simulink model "tanks_with_costate_equations_model"  (R2014a)
settings: Solver=ode4  StartTime=0.0  StopTime=T  FixedStep=0.001  RelTol=1e-3
values from neighbouring files (symbols this model uses):
  a = 31    [tanks_runner.m]
  b = 40    [tanks_runner.m]
  c = 10    [tanks_runner.m]
  C1 = 25    [tanks_runner.m]
  C2 = 25    [tanks_runner.m]
  C3 = 25    [tanks_runner.m]
  h10 = 10    [tanks_runner.m]
  h20 = 10    [tanks_runner.m]
  h30 = 10    [tanks_runner.m]
  h_max = 40    [tanks_runner.m]
  p = [sin(theta)*cos(phi); sin(theta)*sin(phi); cos(theta)]    [tanks_reachability_set.m]
  R = 40    [tanks_runner.m]
  u_max = 200    [tanks_runner.m]
  w = 5    [tanks_runner.m]
settings Model: Creator=Lukasz  LastModifiedBy=Lukasz

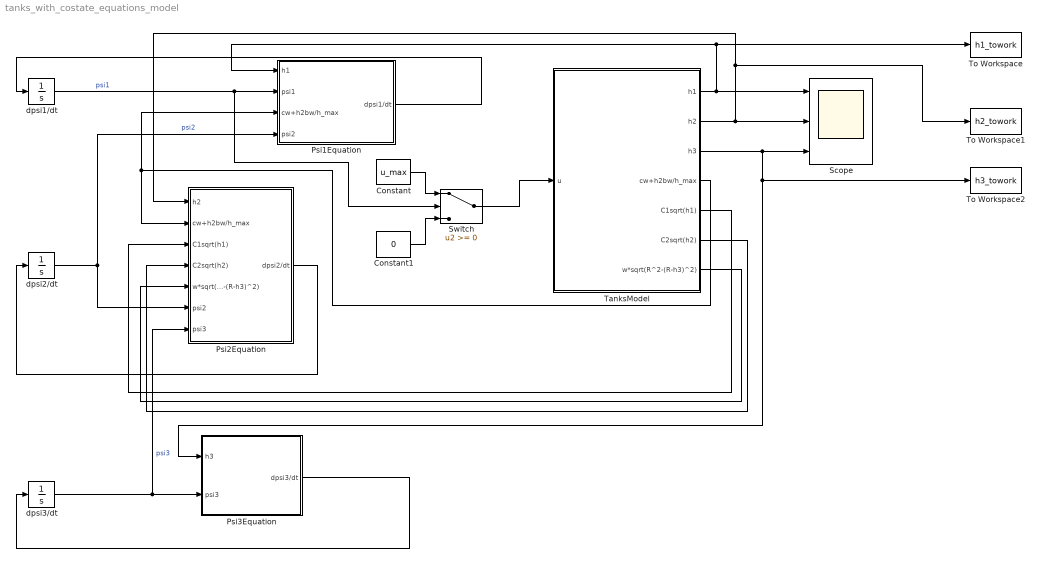
== system tanks_with_costate_equations_model ==
  Constant : Constant  Value=u_max
  Constant1 : Constant  Value=0
  Psi1Equation : Subsystem
  Psi2Equation : Subsystem
  Psi3Equation : Subsystem
  Scope : Scope  NumInputPorts=3
      settings: ShowLegends=on  YMin=-0~-5~-5  YMax=40~5~5  SampleInput=on
  Switch : Switch
  TanksModel : Subsystem
  To Workspace : ToWorkspace  VariableName=h1_towork  SaveFormat=Timeseries  SampleTime=-1
  To Workspace1 : ToWorkspace  VariableName=h2_towork  SaveFormat=Timeseries  SampleTime=-1
  To Workspace2 : ToWorkspace  VariableName=h3_towork  SaveFormat=Timeseries  SampleTime=-1
  dpsi1/dt : Integrator  InitialCondition=p(1)
  dpsi2/dt : Integrator  InitialCondition=p(2)
  dpsi3/dt : Integrator  InitialCondition=p(3)
  wires:
  TanksModel/2(h2) -> To Workspace1/1, Psi2Equation/1(h2), Scope/2
  TanksModel/3(h3) -> Scope/3, Psi3Equation/1(h3), To Workspace2/1
  TanksModel/4("cw+h2bw/h_max ") -> Psi1Equation/3(cw+h2bw/h_max), Psi2Equation/2(cw+h2bw/h_max)
  dpsi1/dt/1 -> Switch/2, Psi1Equation/2(psi1)  "psi1"
  dpsi2/dt/1 -> Psi2Equation/6(psi2), Psi1Equation/4(psi2)  "psi2"
  Psi1Equation/1(dpsi1/dt) -> dpsi1/dt/1
  TanksModel/5(C1sqrt(h1)) -> Psi2Equation/3(C1sqrt(h1))
  TanksModel/6(C2sqrt(h2)) -> Psi2Equation/4(C2sqrt(h2))
  TanksModel/7(w*sqrt(R^2-(R-h3)^2)) -> Psi2Equation/5(w*sqrt(R^2-(R-h3)^2))
  dpsi3/dt/1 -> Psi3Equation/2(psi3), Psi2Equation/7(psi3)  "psi3"
  Psi2Equation/1(dpsi2/dt) -> dpsi2/dt/1
  Psi3Equation/1(dpsi3/dt) -> dpsi3/dt/1
  Constant/1 -> Switch/1
  Constant1/1 -> Switch/3
  Switch/1 -> TanksModel/1(u)
  TanksModel/1(h1) -> Scope/1, To Workspace/1, Psi1Equation/1(h1)

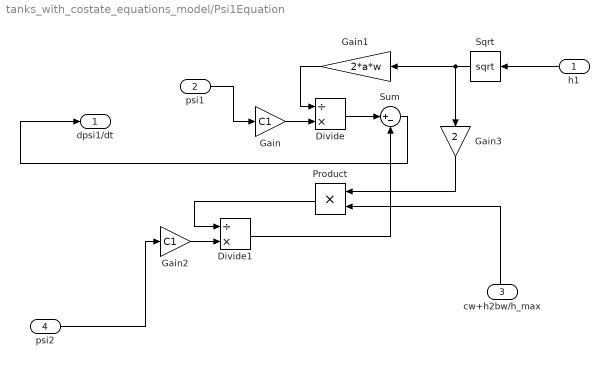
== system tanks_with_costate_equations_model/Psi1Equation ==
  h1 : Inport
  psi1 : Inport  Port=2
  cw+h2bw/h_max : Inport  Port=3
  psi2 : Inport  Port=4
  Divide : Product  Inputs=/*
  Divide1 : Product  Inputs=/*
  Gain : Gain  Gain=C1
  Gain1 : Gain  Gain=2*a*w
  Gain2 : Gain  Gain=C1
  Gain3 : Gain  Gain=2
  Product : Product
  Sqrt : Sqrt  SaturateOnIntegerOverflow=on
  Sum : Sum  Inputs=|+-
  dpsi1/dt : Outport
  wires:
  h1/1 -> Sqrt/1
  cw+h2bw/h_max/1 -> Product/2
  psi2/1 -> Gain2/1
  Product/1 -> Divide1/1
  Divide/1 -> Sum/1
  Sum/1 -> dpsi1/dt/1
  Gain/1 -> Divide/2
  Gain2/1 -> Divide1/2
  Gain1/1 -> Divide/1
  Gain3/1 -> Product/1
  Divide1/1 -> Sum/2
  psi1/1 -> Gain/1
  Sqrt/1 -> Gain1/1, Gain3/1

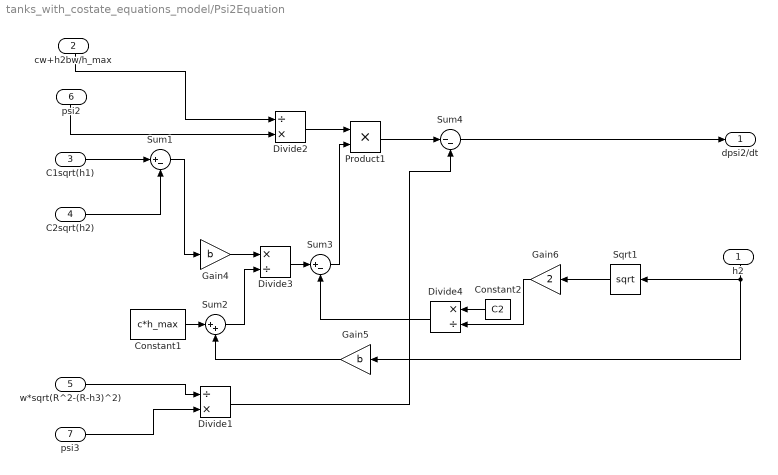
== system tanks_with_costate_equations_model/Psi2Equation ==
  h2 : Inport
  cw+h2bw/h_max : Inport  Port=2
  C1sqrt(h1) : Inport  Port=3
  C2sqrt(h2) : Inport  Port=4
  w*sqrt(R^2-(R-h3)^2) : Inport  Port=5
  psi2 : Inport  Port=6
  psi3 : Inport  Port=7
  Constant1 : Constant  Value=c*h_max
  Constant2 : Constant  Value=C2
  Divide1 : Product  Inputs=/*
  Divide2 : Product  Inputs=/*
  Divide3 : Product  Inputs=*/
  Divide4 : Product  Inputs=*/
  Gain4 : Gain  Gain=b
  Gain5 : Gain  Gain=b
  Gain6 : Gain  Gain=2
  Product1 : Product
  Sqrt1 : Sqrt  SaturateOnIntegerOverflow=on
  Sum1 : Sum  Inputs=|+-
  Sum2 : Sum  Inputs=|++
  Sum3 : Sum  Inputs=|+-
  Sum4 : Sum  Inputs=|--
  dpsi2/dt : Outport
  wires:
  Constant1/1 -> Sum2/1
  Gain5/1 -> Sum2/2
  w*sqrt(R^2-(R-h3)^2)/1 -> Divide1/1
  Product1/1 -> Sum4/1
  psi2/1 -> Divide2/2
  cw+h2bw/h_max/1 -> Divide2/1
  h2/1 -> Gain5/1, Sqrt1/1
  Sqrt1/1 -> Gain6/1
  Sum1/1 -> Gain4/1
  Divide1/1 -> Sum4/2
  Gain6/1 -> Divide4/2
  Sum4/1 -> dpsi2/dt/1
  Divide4/1 -> Sum3/2
  psi3/1 -> Divide1/2
  Sum2/1 -> Divide3/2
  Gain4/1 -> Divide3/1
  Divide2/1 -> Product1/1
  Divide3/1 -> Sum3/1
  Sum3/1 -> Product1/2
  Constant2/1 -> Divide4/1
  C1sqrt(h1)/1 -> Sum1/1
  C2sqrt(h2)/1 -> Sum1/2

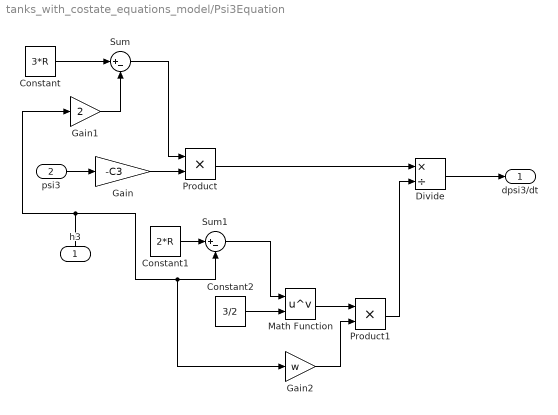
== system tanks_with_costate_equations_model/Psi3Equation ==
  h3 : Inport
  psi3 : Inport  Port=2
  Constant : Constant  Value=3*R
  Constant1 : Constant  Value=2*R
  Constant2 : Constant  Value=3/2
  Divide : Product  Inputs=*/
  Gain : Gain  Gain=-C3
  Gain1 : Gain  Gain=2
  Gain2 : Gain  Gain=w
  Math Function : Math  Operator=pow  SaturateOnIntegerOverflow=on
  Product : Product
  Product1 : Product
  Sum : Sum  Inputs=|+-
  Sum1 : Sum  Inputs=|+-
  dpsi3/dt : Outport
  wires:
  Constant/1 -> Sum/1
  Divide/1 -> dpsi3/dt/1
  Product1/1 -> Divide/2
  Product/1 -> Divide/1
  Constant2/1 -> Math Function/2
  Math Function/1 -> Product1/1
  Gain1/1 -> Sum/2
  Sum/1 -> Product/1
  Sum1/1 -> Math Function/1
  Constant1/1 -> Sum1/1
  Gain2/1 -> Product1/2
  h3/1 -> Gain2/1, Sum1/2, Gain1/1
  psi3/1 -> Gain/1
  Gain/1 -> Product/2

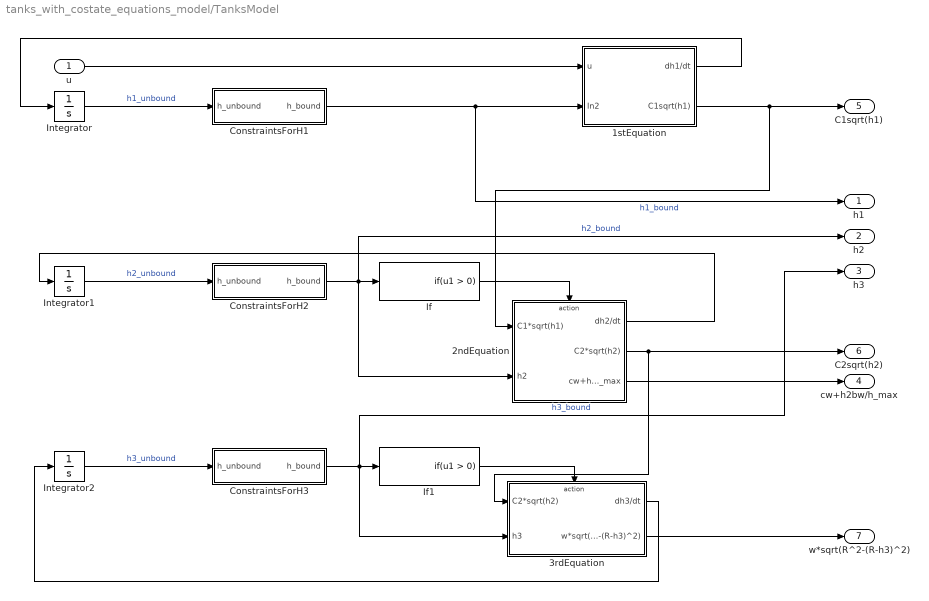
== system tanks_with_costate_equations_model/TanksModel ==
  u : Inport
  1stEquation : Subsystem
  2ndEquation : Subsystem
  3rdEquation : Subsystem
  ConstraintsForH1 : Subsystem
  ConstraintsForH2 : Subsystem
  ConstraintsForH3 : Subsystem
  If : If  ShowElse=off
  If1 : If  ShowElse=off
  Integrator : Integrator  InitialCondition=h10
  Integrator1 : Integrator  InitialCondition=h20
  Integrator2 : Integrator  InitialCondition=h30
  h1 : Outport
  h2 : Outport  Port=2
  h3 : Outport  Port=3
  "cw+h2bw/h_max " : Outport  Port=4
  C1sqrt(h1) : Outport  Port=5
  C2sqrt(h2) : Outport  Port=6
  w*sqrt(R^2-(R-h3)^2) : Outport  Port=7
  wires:
  Integrator1/1 -> ConstraintsForH2/1(h_unbound)  "h2_unbound"
  Integrator2/1 -> ConstraintsForH3/1(h_unbound)  "h3_unbound"
  ConstraintsForH1/1(h_bound) -> h1/1, 1stEquation/2(In2)  "h1_bound"
  Integrator/1 -> ConstraintsForH1/1(h_unbound)  "h1_unbound"
  ConstraintsForH2/1(h_bound) -> If/1, 2ndEquation/2(h2), h2/1  "h2_bound"
  ConstraintsForH3/1(h_bound) -> If1/1, 3rdEquation/2(h3), h3/1  "h3_bound"
  2ndEquation/1(dh2/dt) -> Integrator1/1
  If/1 -> 2ndEquation/Action
  2ndEquation/2(C2*sqrt(h2)) -> C2sqrt(h2)/1, 3rdEquation/1(C2*sqrt(h2))
  3rdEquation/1(dh3/dt) -> Integrator2/1
  u/1 -> 1stEquation/1(u)
  1stEquation/1(dh1/dt) -> Integrator/1
  1stEquation/2(C1sqrt(h1)) -> C1sqrt(h1)/1, 2ndEquation/1(C1*sqrt(h1))
  2ndEquation/3(cw+h2bw/h_max) -> "cw+h2bw/h_max "/1
  If1/1 -> 3rdEquation/Action
  3rdEquation/2(w*sqrt(R^2-(R-h3)^2)) -> w*sqrt(R^2-(R-h3)^2)/1

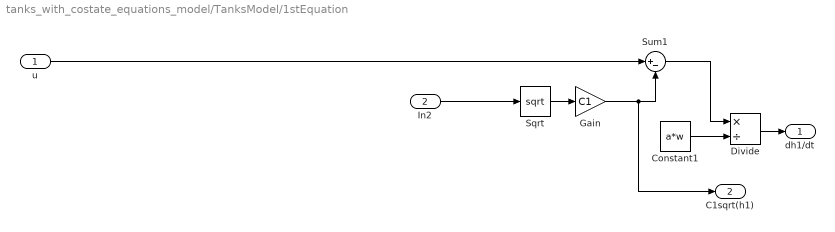
== system tanks_with_costate_equations_model/TanksModel/1stEquation ==
  u : Inport
  In2 : Inport  Port=2
  Constant1 : Constant  Value=a*w
  Divide : Product  Inputs=*/
  Gain : Gain  Gain=C1
  Sqrt : Sqrt  SaturateOnIntegerOverflow=on
  Sum1 : Sum  Inputs=|+-
  dh1/dt : Outport
  C1sqrt(h1) : Outport  Port=2
  wires:
  In2/1 -> Sqrt/1
  Constant1/1 -> Divide/2
  Divide/1 -> dh1/dt/1
  u/1 -> Sum1/1
  Gain/1 -> C1sqrt(h1)/1, Sum1/2
  Sqrt/1 -> Gain/1
  Sum1/1 -> Divide/1

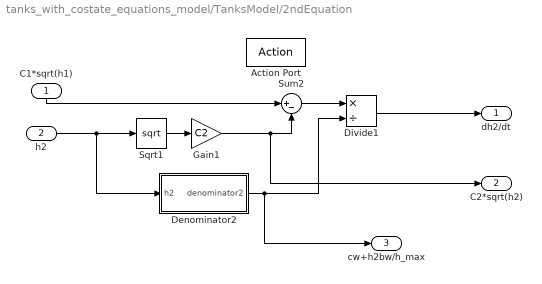
== system tanks_with_costate_equations_model/TanksModel/2ndEquation ==
  C1*sqrt(h1) : Inport
  h2 : Inport  Port=2
  Action Port : ActionPort  ActionType=then
  Denominator2 : Subsystem
  Divide1 : Product  Inputs=*/
  Gain1 : Gain  Gain=C2
  Sqrt1 : Sqrt  SaturateOnIntegerOverflow=on
  Sum2 : Sum  Inputs=|+-
  dh2/dt : Outport
  C2*sqrt(h2) : Outport  Port=2
  cw+h2bw/h_max : Outport  Port=3
  wires:
  Sqrt1/1 -> Gain1/1
  Gain1/1 -> C2*sqrt(h2)/1, Sum2/2
  Denominator2/1(denominator2) -> cw+h2bw/h_max/1, Divide1/2
  Sum2/1 -> Divide1/1
  Divide1/1 -> dh2/dt/1
  h2/1 -> Denominator2/1(h2), Sqrt1/1
  C1*sqrt(h1)/1 -> Sum2/1

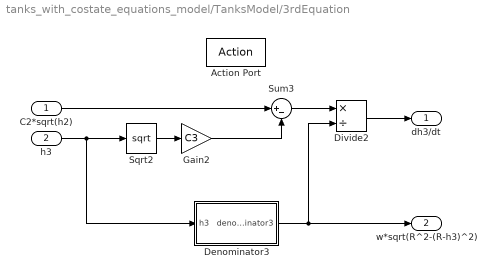
== system tanks_with_costate_equations_model/TanksModel/3rdEquation ==
  C2*sqrt(h2) : Inport
  h3 : Inport  Port=2
  Action Port : ActionPort  ActionType=then
  Denominator3 : Subsystem
  Divide2 : Product  Inputs=*/
  Gain2 : Gain  Gain=C3
  Sqrt2 : Sqrt  SaturateOnIntegerOverflow=on
  Sum3 : Sum  Inputs=|+-
  dh3/dt : Outport
  w*sqrt(R^2-(R-h3)^2) : Outport  Port=2
  wires:
  Sum3/1 -> Divide2/1
  Divide2/1 -> dh3/dt/1
  Sqrt2/1 -> Gain2/1
  Gain2/1 -> Sum3/2
  Denominator3/1(denominator3) -> w*sqrt(R^2-(R-h3)^2)/1, Divide2/2
  C2*sqrt(h2)/1 -> Sum3/1
  h3/1 -> Denominator3/1(h3), Sqrt2/1

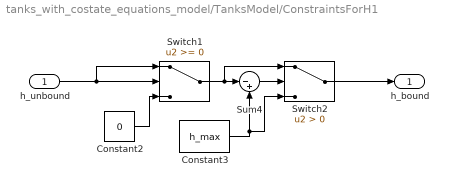
== system tanks_with_costate_equations_model/TanksModel/ConstraintsForH1 ==
  h_unbound : Inport
  Constant2 : Constant  Value=0
  Constant3 : Constant  Value=h_max
  Sum4 : Sum  Inputs=|-+
  Switch1 : Switch
  Switch2 : Switch  Criteria=u2 > Threshold
  h_bound : Outport
  wires:
  h_unbound/1 -> Switch1/2, Switch1/1
  Constant2/1 -> Switch1/3
  Switch1/1 -> Switch2/1, Sum4/1
  Switch2/1 -> h_bound/1
  Sum4/1 -> Switch2/2
  Constant3/1 -> Sum4/2, Switch2/3

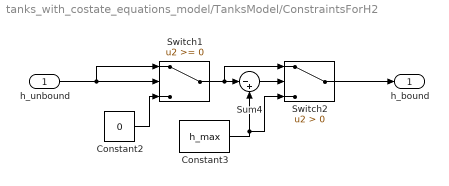
== system tanks_with_costate_equations_model/TanksModel/ConstraintsForH2 ==
  h_unbound : Inport
  Constant2 : Constant  Value=0
  Constant3 : Constant  Value=h_max
  Sum4 : Sum  Inputs=|-+
  Switch1 : Switch
  Switch2 : Switch  Criteria=u2 > Threshold
  h_bound : Outport
  wires:
  Constant3/1 -> Switch2/3, Sum4/2
  Sum4/1 -> Switch2/2
  Switch2/1 -> h_bound/1
  Switch1/1 -> Sum4/1, Switch2/1
  Constant2/1 -> Switch1/3
  h_unbound/1 -> Switch1/1, Switch1/2

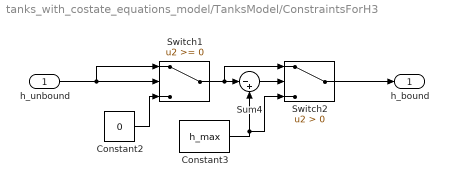
== system tanks_with_costate_equations_model/TanksModel/ConstraintsForH3 ==
  h_unbound : Inport
  Constant2 : Constant  Value=0
  Constant3 : Constant  Value=h_max
  Sum4 : Sum  Inputs=|-+
  Switch1 : Switch
  Switch2 : Switch  Criteria=u2 > Threshold
  h_bound : Outport
  wires:
  h_unbound/1 -> Switch1/2, Switch1/1
  Constant2/1 -> Switch1/3
  Switch1/1 -> Switch2/1, Sum4/1
  Switch2/1 -> h_bound/1
  Sum4/1 -> Switch2/2
  Constant3/1 -> Sum4/2, Switch2/3

== system tanks_with_costate_equations_model/TanksModel/2ndEquation/Denominator2 ==
  h2 : Inport
  Constant : Constant  Value=c*w
  Gain3 : Gain  Gain=b*w/h_max
  Sum : Sum  Inputs=|++
  denominator2 : Outport
  wires:
  Sum/1 -> denominator2/1
  Constant/1 -> Sum/2
  h2/1 -> Gain3/1
  Gain3/1 -> Sum/1

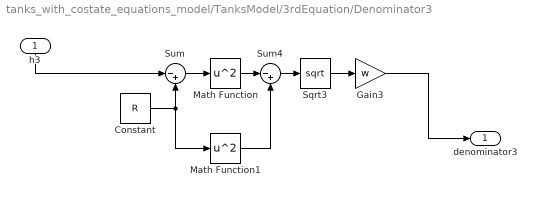
== system tanks_with_costate_equations_model/TanksModel/3rdEquation/Denominator3 ==
  h3 : Inport
  Constant : Constant  Value=R
  Gain3 : Gain  Gain=w
  Math Function : Math  Operator=square  SaturateOnIntegerOverflow=on
  Math Function1 : Math  Operator=square  SaturateOnIntegerOverflow=on
  Sqrt3 : Sqrt  SaturateOnIntegerOverflow=on
  Sum : Sum  Inputs=|-+
  Sum4 : Sum  Inputs=|-+
  denominator3 : Outport
  wires:
  Sum/1 -> Math Function/1
  Sqrt3/1 -> Gain3/1
  Math Function1/1 -> Sum4/2
  Sum4/1 -> Sqrt3/1
  h3/1 -> Sum/1
  Math Function/1 -> Sum4/1
  Gain3/1 -> denominator3/1
  Constant/1 -> Sum/2, Math Function1/1
